simulink model "sim_discreto"  (R2025a)
settings: Solver=FixedStepAuto  StartTime=0.0  StopTime=40  FixedStep=0.001  RelTol=1e-3
libraries: cstblocks x2
settings Model: Creator=danielsaenzobando  LastModifiedBy=danielsaenzobando

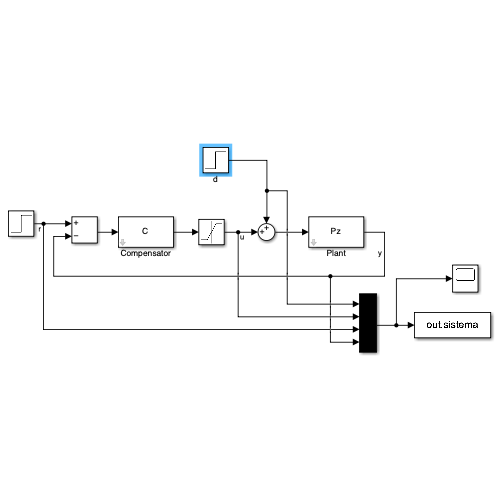
[thumbnail: Simulink's stored preview of the top-level diagram]
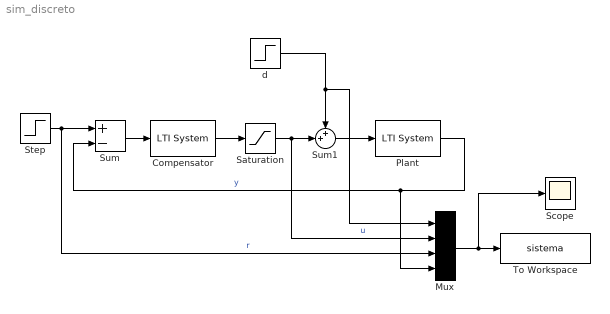
== system sim_discreto ==
  Compensator : cstblocks/LTI System  sys=C  IC=[]  PadeOrder=0
  Mux : Mux
  Plant : cstblocks/LTI System  sys=Pz  IC=[]  PadeOrder=0
  Saturation : Saturate  UpperLimit=100  LowerLimit=0
  Scope : Scope
      settings: ActiveDisplayYMinimum=13.318850267379673  ActiveDisplayYMaximum=24.515374331550802
  Step : Step  Time=5  After=20  SampleTime=0
  Sum : Sum  Inputs=+-
  Sum1 : Sum  Inputs=++|
  To Workspace : ToWorkspace  VariableName=sistema  SaveFormat=Timeseries  SampleTime=-1
  d : Step  Time=20  After=10  SampleTime=0
  wires:
  Step/1 -> Mux/3, Sum/1  "r"
  Sum/1 -> Compensator/1
  Plant/1 -> Mux/4, Sum/2  "y"
  d/1 -> Mux/1, Sum1/1
  Sum1/1 -> Plant/1
  Compensator/1 -> Saturation/1
  Saturation/1 -> Mux/2, Sum1/2  "u"
  Mux/1 -> Scope/1, To Workspace/1
